simulink model "UDP_INTEGRATION_TEST_01"  (Simulink 8.1)
settings: Solver=ode4  StartTime=0.0  StopTime=inf  FixedStep=Ts  MaxStep=1e-3  RelTol=1e-3
model workspace (MAT data in the model file):
  op_snapshot1 : opcond.OperatingPoint (value not decoded)
PostLoadFcn:
  | INTEGRATION_TEST_01_init;
InitFcn:
  | INTEGRATION_TEST_01_init;
undefined symbols (not defined in the file or in its folder): cable_spec, fdesignblkfcn, gcbh, generic_ethernet_cb, Left, relay_par, Ts, type, V
libraries: powerlib_extras x14, rtio_opalrt_common x13, rtlab x10, cables_lib x6, breaker_lib x4, simulink_extras x4, simulink x4, Load_lib x3, rtio_generic_modbus x3, powerlib x2, ssn_lib x2, transformer_lib x2
(part 1 of 2)
settings Model: ARTEMISmethode_block_infos=$$__separator__$$UDP_INTEGRATION_TEST_01/ARTEMIS Guide$$__separator__$$  Creator=RE25624  LastModifiedBy=re25624  BufferReuse=off
settings SolverCC: ZeroCrossAlgorithm=Adaptive
settings DataIOCC: ExternalInput=getinputstruct(op_snapshot1)  InitialState=getstatestruct(op_snapshot1)  LimitDataPoints=off  MaxDataPoints=90060  SignalLoggingSaveFormat=Dataset  SaveOutput=off  SignalLogging=off  DSMLogging=off  SaveTime=off  OutputSaveName=result
settings OptimizationCC: BlockReduction=off  OptimizeBlockIOStorage=off  BufferReuse=off  ExpressionFolding=off  LocalBlockOutputs=off
settings DebuggingCC: MaxConsecutiveZCsMsg=warning  IgnoredZcDiagnostic=none  SolverPrmCheckMsg=none  MultiTaskRateTransMsg=warning  FcnCallInpInsideContextMsg=EnableAllAsWarning  FrameProcessingCompatibilityMsg=error  ModelReferenceExtraNoncontSigs=warning  StrictBusMsg=None
settings ModelReferenceCC: UpdateModelReferenceTargets=IfOutOfDate
settings SFSimCC: SFSimEcho=off
settings GRTTargetCC: CodeReplacementLibrary=C89/C90 (ANSI)

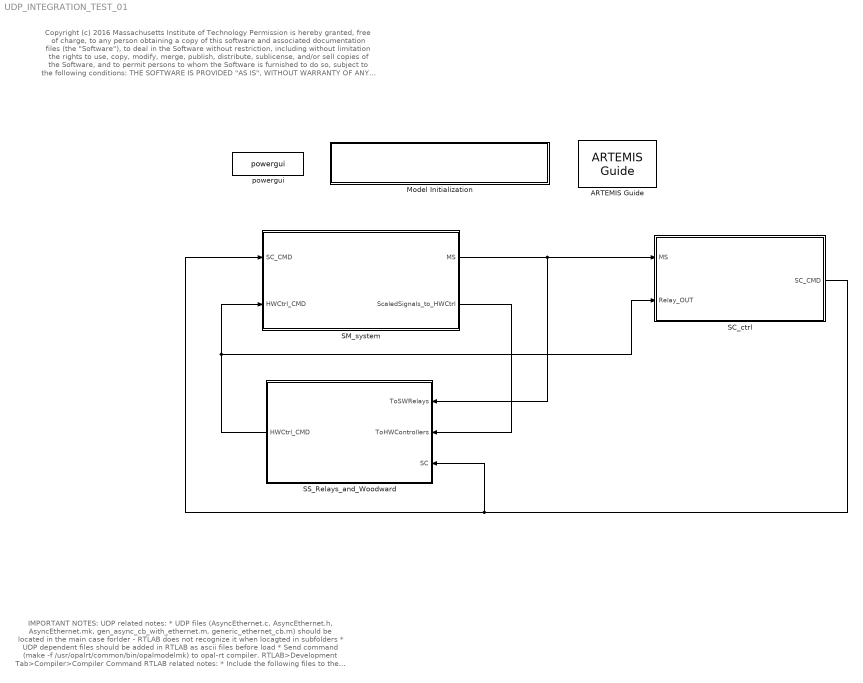
== system UDP_INTEGRATION_TEST_01 ==
  note: Copyright (c) 2016 Massachusetts Institute of Technology
      | Permission is hereby granted, free of charge, to any person obtaining a copy of this software and associated documentation files (the "Software"), to deal
      | in the Software without restriction, including without limitation the rights to use, copy, modify, merge, publish, distribute, sublicense, and/or sell copies of the
      | Software, and to permit persons to whom the Software is furnished to do so, subject to the following conditions:
      |
      | THE SOFTWARE IS PROVIDED "AS IS", WITHOUT WARRANTY OF ANY KIND, EXPRESS OR IMPLIED, INCLUDING BUT NOT LIMITED TO THE
      | WARRANTIES OF MERCHANTABILITY, FITNESS FOR A PARTICULAR PURPOSE AND NONINFRINGEMENT. IN NO EVENT SHALL THE AUTHORS
      | OR COPYRIGHT HOLDERS BE LIABLE FOR ANY CLAIM, DAMAGES OR OTHER LIABILITY, WHETHER IN AN ACTION OF CONTRACT, TORT OR
      | OTHERWISE, ARISING FROM, OUT OF OR IN CONNECTION WITH THE SOFTWARE OR THE USE OR OTHER DEALINGS IN THE SOFTWARE.
  note: IMPORTANT NOTES:
      |
      | UDP related notes:
      | * UDP files (AsyncEthernet.c, AsyncEthernet.h, AsyncEthernet.mk, gen_async_cb_with_ethernet.m, generic_ethernet_cb.m)
      | should be located in the main case forlder - RTLAB does not recognize it when locagted in subfolders
      | * UDP dependent files should be added in RTLAB as ascii files before load
      | * Send command (make -f /usr/opalrt/common/bin/opalmodelmk) to opal-rt compiler.   RTLAB>Development Tab>Compiler>Compiler Command
      |
      | RTLAB related notes:
      | * Include the following files to the case before compilation:
      | ascii (..\..\..\..\..\Program Files (x86)\MATLAB\R2013a\toolbox\physmod\powersys\powersys\sfun_discreteVariableDelay.c)
      | binary (..\..\..\..\..\Program Files (x86)\MATLAB\R2013a\toolbox\physmod\powersys\powersys\sfun_discreteVariableDelay.mexw32)
  ARTEMIS Guide : artemis/ARTEMIS/ARTEMIS Guide  Tag=FTSSmethode_opal_4hx0r99  Description=5.0_z1  lock=on  Ts=Ts  opt=art5  dyna=off  nb_perm=4  RT_fullcomp=off  ssn=on  ssn_itvc=off  ssn_ivic=off  ssn_ext=off  ssn_solver=Art5 with Backward Euler nodal interface  ssn_impulse=off  ssn_quasimpulse=off  ssn_impulse_loop=2  paraExtinctionThy=off  Thy_Impulse=on  dtc=Off  dtc_opt=normal  ao=on  simtype=off  ct_mac=off  lin_mov=off  lsp=[0.001 2]  spike_skip=Disabled  dtc_extra=1  dtc_sws=normal  dtc_pied=0.5  SPSRulesBlock=SPSRules  tre=on  ctmm=off  LF=off  dpl_type=ARTEMiS DPL  rlc_type=off  custom_type=off  para=on  ssn_ImpulseLoopBlockedStateUpdate=2  ssn_mov_iter_number=5  ssn_switch_iter_number=5
  Model Initialization : Subsystem  AncestorBlock=artemis/Tools /Misc/Model Initialization  mask(Model Functions){InitFcnX=INTEGRATION_TEST_01_init;, prel=off, posl=on, inif=on, strf=off}
      mask prompts: InitFcnX "Initialisation"; prel "Preload Function"; posl "PostLoad Function"; inif "InitFcn"; strf "StartFcn"
      mask init:
      | currentBlock = gcb;
      | root = bdroot(currentBlock);
      | 
      | 
      | if ~strcmp(get_param(root,'BlockDiagramType'),'library')
      |     if prel==1
      |         set_param(root, 'PreLoadFcn', InitFcnX);
      |     else
      |         set_param(root, 'PreLoadFcn', '');
      |     end
      |     if inif==1
      |         set_param(root, 'InitFcn', InitFcnX);
      |     else
      |         set_param(root, 'InitFcn', '');
      |     end
      |     if strf==1
      |         set_param(root, 'StartFcn', InitFcnX);
      |     else
      |         set_param(root, 'StartFcn', '');
      |     end
      |     if posl==1
      |         set_param(root, 'PostLoadFcn', InitFcnX);
      |     else
      |         set_param(root, 'PostLoadFcn', '');
      |     end
      | end
      | 
      | pos = get_param(currentBlock, 'Position');
      | width = pos(3) - pos(1); height = pos(4) - pos(2);
      | txt = [ upper(root) '\n' '- InitFcn. . . . . '  get_param(root, 'InitFcn') ];
      settings: CopyFcn=set_param(gcb,'LinkStatus','inactive')
      mask Display: text(5, height*0.5, txt, 'horizontalAlignment', 'left', 'verticalAlignment', 'middle') ;
  SC_ctrl : Subsystem
  SM_system : Subsystem
  SS_Relays_and_Woodward : Subsystem
  powergui : powerlib/powergui  Priority=2  SimulationMode=Discrete  SolverType=Tustin  SampleTime=Ts  frequency=60  SPID=off  DisableSnubberDevices=off  DisableRonSwitches=off  DisableVfSwitches=off  SwTol=0  Interpol=off  DisplayEquations=off  frequencyindice=0  Pbase=100e6  ErrMax=1e-4  Iterations=50  UnitsV=kV  UnitsW=MW  FunctionMessages=off  echomessages=off  HookPort=off  EnableUseOfTLC=off  x0status=blocks  RestoreLinks=warning  ResistiveCurrentMeasurement=off  Frange=logspace(0,3,50)  Ylog=off  Xlog=off  ShowGrid=off  save=off  variable=ZData  structure=0  ZoomFFT=on  StartTime=0.0  cycles=2  DisplayStyle=off  fundamental=60  FreqAxis=off  MaxFrequency=1000  frequencyindicesteady=1  RmsSteady=1  display=off  Ts=0  methode=off
  wires:
  SS_Relays_and_Woodward/1(HWCtrl_CMD) -> SM_system/2(HWCtrl_CMD), SC_ctrl/2(Relay_OUT)
  SC_ctrl/1(SC_CMD) -> SS_Relays_and_Woodward/3(SC), SM_system/1(SC_CMD)
  SM_system/1(MS) -> SC_ctrl/1(MS), SS_Relays_and_Woodward/1(ToSWRelays)
  SM_system/2(ScaledSignals_to_HWCtrl) -> SS_Relays_and_Woodward/2(ToHWControllers)

== system UDP_INTEGRATION_TEST_01/Model Initialization ==

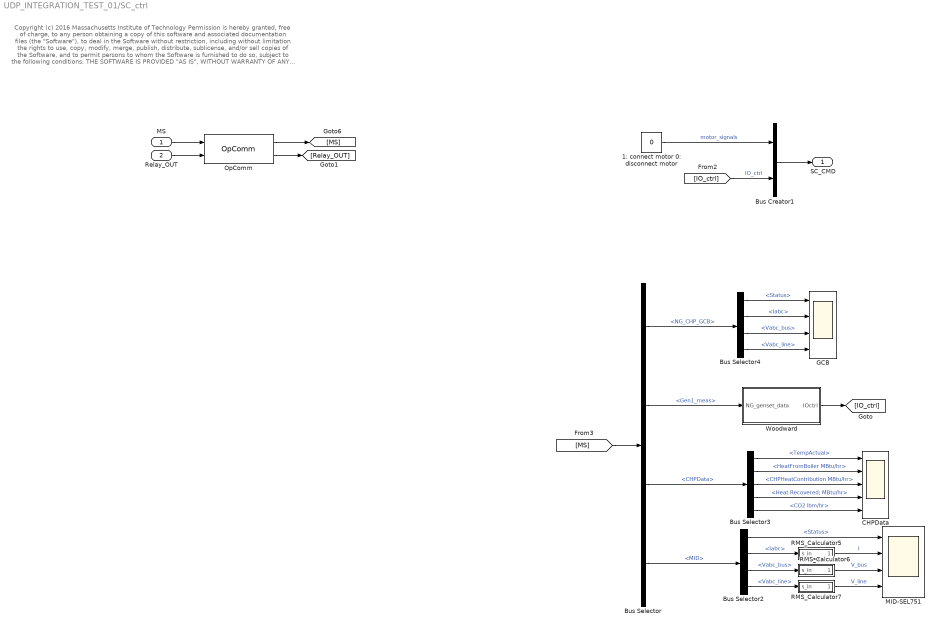
== system UDP_INTEGRATION_TEST_01/SC_ctrl ==
  note: Copyright (c) 2016 Massachusetts Institute of Technology
      | Permission is hereby granted, free of charge, to any person obtaining a copy of this software and associated documentation files (the "Software"), to deal
      | in the Software without restriction, including without limitation the rights to use, copy, modify, merge, publish, distribute, sublicense, and/or sell copies of the
      | Software, and to permit persons to whom the Software is furnished to do so, subject to the following conditions:
      |
      | THE SOFTWARE IS PROVIDED "AS IS", WITHOUT WARRANTY OF ANY KIND, EXPRESS OR IMPLIED, INCLUDING BUT NOT LIMITED TO THE
      | WARRANTIES OF MERCHANTABILITY, FITNESS FOR A PARTICULAR PURPOSE AND NONINFRINGEMENT. IN NO EVENT SHALL THE AUTHORS
      | OR COPYRIGHT HOLDERS BE LIABLE FOR ANY CLAIM, DAMAGES OR OTHER LIABILITY, WHETHER IN AN ACTION OF CONTRACT, TORT OR
      | OTHERWISE, ARISING FROM, OUT OF OR IN CONNECTION WITH THE SOFTWARE OR THE USE OR OTHER DEALINGS IN THE SOFTWARE
  MS : Inport
  Relay_OUT : Inport  Port=2
  1: connect motor 0: disconnect motor : Constant  Value=0
  Bus Creator1 : BusCreator  Inputs=2
  Bus Selector : BusSelector  OutputSignals=NG_CHP_MS.NG_CHP_GCB,NG_CHP_MS.Gen1_meas,NG_CHP_MS.CHPData,MID
  Bus Selector2 : BusSelector  OutputSignals=Status,Iabc,Vabc_bus,Vabc_line
  Bus Selector3 : BusSelector  OutputSignals=TempActual,HeatFromBoiler MBtu/hr,CHPHeatContribution MBtu/hr,Thermal data.Heat Recovered; MBtu/hr,Thermal data.CO2 lbm/hr
  Bus Selector4 : BusSelector  OutputSignals=Status,Iabc,Vabc_bus,Vabc_line
  CHPData : Scope  NumInputPorts=5
      settings: ShowLegends=on  TimeRange=10  YMin=19.11~0~-1~1.37518~932.98  YMax=19.2~5.5~1~1.37533~933.08  SaveName=ScopeData3
  GCB : Scope  NumInputPorts=4
      settings: ShowLegends=on  TimeRange=1  YMin=-1~-0.001~-12000~-12000  YMax=1~0.001~12000~12000  SaveName=ScopeData6
  MID-SEL751 : Scope  NumInputPorts=4
      settings: ShowLegends=on  TimeRange=1  YMin=0.95~-225~-12000~-12000  YMax=1.05~225~12000~12000  SaveName=ScopeData9
  OpComm : rtlab/OpComm  nbport=2  groupe_acq=1  subsys_rate=0  st=0  Synchronization=on  Interpolation=on  Threshold=1.0  Missed_Data=off  Sim_Time=off  Samples=off  dynSigOut=off  from_console=0  warning_done=off  writeOpCommFile=off  Offset=off
  RMS_Calculator5 : Subsystem
  RMS_Calculator6 : Subsystem
  RMS_Calculator7 : Subsystem
  Woodward : Subsystem
  SC_CMD : Outport
  wires:
  OpComm/1 -> [MS]
  MS/1 -> OpComm/1
  OpComm/2 -> [Relay_OUT]
  Relay_OUT/1 -> OpComm/2
  [IO_ctrl] -> Bus Creator1/2  "IO_ctrl"
  1: connect motor 0: disconnect motor/1 -> Bus Creator1/1  "motor_signals"
  Bus Creator1/1 -> SC_CMD/1
  Bus Selector/4 -> Bus Selector2/1  "<MID>"
  RMS_Calculator7/1(s_out) -> MID-SEL751/4  "V_line"
  RMS_Calculator6/1(s_out) -> MID-SEL751/3  "V_bus"
  RMS_Calculator5/1(s_out) -> MID-SEL751/2  "I"
  Bus Selector2/4 -> RMS_Calculator7/1(s_in)  "<Vabc_line>"
  Bus Selector2/3 -> RMS_Calculator6/1(s_in)  "<Vabc_bus>"
  Bus Selector2/2 -> RMS_Calculator5/1(s_in)  "<Iabc>"
  Bus Selector2/1 -> MID-SEL751/1  "<Status>"
  Bus Selector3/4 -> CHPData/4  "<Heat Recovered; MBtu/hr>"
  Bus Selector3/3 -> CHPData/3  "<CHPHeatContribution MBtu/hr>"
  Bus Selector3/2 -> CHPData/2  "<HeatFromBoiler MBtu/hr>"
  Bus Selector3/5 -> CHPData/5  "<CO2 lbm/hr>"
  Bus Selector3/1 -> CHPData/1  "<TempActual>"
  Bus Selector/3 -> Bus Selector3/1  "<CHPData>"
  [MS] -> Bus Selector/1
  Bus Selector/2 -> Woodward/1(NG_genset_data)  "<Gen1_meas>"
  Bus Selector/1 -> Bus Selector4/1  "<NG_CHP_GCB>"
  Bus Selector4/4 -> GCB/4  "<Vabc_line>"
  Bus Selector4/3 -> GCB/3  "<Vabc_bus>"
  Bus Selector4/2 -> GCB/2  "<Iabc>"
  Bus Selector4/1 -> GCB/1  "<Status>"
  Woodward/1(IOctrl) -> [IO_ctrl]

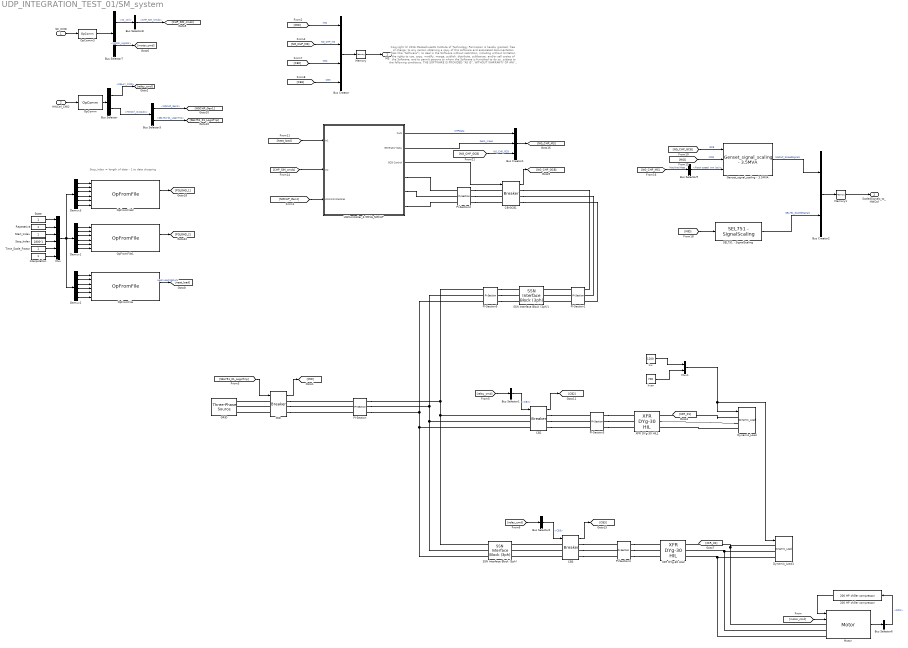
== system UDP_INTEGRATION_TEST_01/SM_system ==
  note: Copyright (c) 2016 Massachusetts Institute of Technology
      | Permission is hereby granted, free of charge, to any person obtaining a copy of this software and associated documentation files (the "Software"), to deal
      | in the Software without restriction, including without limitation the rights to use, copy, modify, merge, publish, distribute, sublicense, and/or sell copies of the
      | Software, and to permit persons to whom the Software is furnished to do so, subject to the following conditions:
      |
      | THE SOFTWARE IS PROVIDED "AS IS", WITHOUT WARRANTY OF ANY KIND, EXPRESS OR IMPLIED, INCLUDING BUT NOT LIMITED TO THE
      | WARRANTIES OF MERCHANTABILITY, FITNESS FOR A PARTICULAR PURPOSE AND NONINFRINGEMENT. IN NO EVENT SHALL THE AUTHORS
      | OR COPYRIGHT HOLDERS BE LIABLE FOR ANY CLAIM, DAMAGES OR OTHER LIABILITY, WHETHER IN AN ACTION OF CONTRACT, TORT OR
      | OTHERWISE, ARISING FROM, OUT OF OR IN CONNECTION WITH THE SOFTWARE OR THE USE OR OTHER DEALINGS IN THE SOFTWARE
  note: Stop_index = length of data - 1 to data chopping
  SC_CMD : Inport
  HWCtrl_CMD : Inport  Port=2
  200 HP chiller compressor : Load_lib/200 HP chiller compressor
  Bus Creator : BusCreator
  Bus Creator1 : BusCreator  Inputs=3
  Bus Creator2 : BusCreator  Inputs=2
  Bus Selector : BusSelector  OutputSignals=RELAY_CMD,HWCtrl_Outputs
  Bus Selector1 : BusSelector  OutputSignals=CB2
  Bus Selector2 : BusSelector  OutputSignals=CB3
  Bus Selector3 : BusSelector  OutputSignals=NGCHP_Gen1,SEL751-01_LogicTrip
  Bus Selector6 : BusSelector  OutputSignals=RPM
  Bus Selector7 : BusSelector  OutputSignals=IO_ctrl,motor_signals
  Bus Selector8 : BusSelector  OutputSignals=16 DOUT GR3.CHP_SIM_Cmds
  Bus Selector9 : BusSelector  OutputSignals="Gen1_meas.w.w.Rotor speed  wm (pu)"
  CB-GCB1 : breaker_lib/Breaker  Ts=Ts  mech_delay=cb_mech_delay
  CB2 : breaker_lib/Breaker  Ts=Ts  mech_delay=cb_mech_delay
  CB3 : breaker_lib/Breaker  Ts=Ts  mech_delay=cb_mech_delay
  Demux1 : Demux  Outputs=6
  Demux2 : Demux  Outputs=6
  Demux3 : Demux  Outputs=6
  Dynamic_Load : Load_lib/Dynamic_Load  V=480  Ts=Ts
  Dynamic_Load1 : Load_lib/Dynamic_Load  V=480  Ts=Ts
  GRID : powerlib/Electrical Sources/Three-Phase Source  Voltage=13800  PhaseAngle=0  Frequency=60  InternalConnection=Yg  SpecifyImpedance=on  Resistance=0.8929  Inductance=16.58e-3  ShortCircuitLevel=375e6  BaseVoltage=13800  XRratio=4.6  BusType=swing  Pref=0  Qref=0  Qmin=-inf  Qmax=inf
  Genset_signal_scaling - 3.5MVA : EasyGen3500_GensetSignalScaling_lib/Genset_signal_scaling - 3.5MVA  Vpk_mcb=11268  watt_mcb=3150000  Vpk_gcb=11268  watt_gcb=3150000  rated_rpm=1800  wm_noise_bias=0.02
  HWController_3.5MVA_NGCHP : Subsystem  AncestorBlock=HWController_NGCHP_Genset_3p5MVA_lib/HWController_3.5MVA_NGCHP
  "Interpolation " : Constant
  MID : breaker_lib/Breaker  Ts=Ts  mech_delay=cb_mech_delay
  Memory : Memory
  Memory1 : Memory
  Motor : Motor_InductionMachine_lib/Motor
  Mux : Mux  Inputs=6
  Mux1 : Mux  Inputs=2
  OpComm : rtlab/OpComm  nbport=1  groupe_acq=1  subsys_rate=0  st=0  Synchronization=on  Interpolation=on  Threshold=1.0  Missed_Data=off  Sim_Time=off  Samples=off  dynSigOut=off  from_console=0  warning_done=off  writeOpCommFile=off  Offset=off
  OpComm3 : rtlab/OpComm  nbport=1  groupe_acq=1  subsys_rate=0  st=0  Synchronization=on  Interpolation=on  Threshold=1.0  Missed_Data=off  Sim_Time=off  Samples=off  dynSigOut=off  from_console=1  warning_done=off  writeOpCommFile=off  Offset=off
  OpFromFile : rtlab/DataLogging/OpFromFile  filename_mode=Static (same filename all the time)  reload_mode=Next time model is paused (Real-Time)  init_file_id=0  filename=HeatLoad.mat  rtpath='./'  nrtpath='.\'  sample_time=Ts
  OpFromFile1 : rtlab/DataLogging/OpFromFile  filename_mode=Static (same filename all the time)  reload_mode=Next time model is paused (Real-Time)  init_file_id=0  filename=one_min_data.mat  rtpath='./'  nrtpath='.\'  sample_time=0
  OpFromFile2 : rtlab/DataLogging/OpFromFile  filename_mode=Static (same filename all the time)  reload_mode=Next time model is paused (Real-Time)  init_file_id=0  filename=one_min_data.mat  rtpath='./'  nrtpath='.\'  sample_time=0
  PI-Section : cables_lib/PI-Section  cable_spec=[cable_spec(13, :)]  line_length=5500  parallel_sets=2
  PI-Section1 : cables_lib/PI-Section  cable_spec=[cable_spec(11, :)]  line_length=10  parallel_sets=1
  PI-Section2 : cables_lib/PI-Section  cable_spec=[cable_spec(11, :)]  line_length=2000  parallel_sets=1
  PI-Section3 : cables_lib/PI-Section  cable_spec=[cable_spec(13, :)]  line_length=1500  parallel_sets=1
  PI-Section4 : cables_lib/PI-Section  cable_spec=[cable_spec(13, :)]  line_length=2000  parallel_sets=2
  PI-Section5 : cables_lib/PI-Section  cable_spec=[cable_spec(11, :)]  line_length=10  parallel_sets=1
  "Repetative " : Constant
  SEL751 - SignalScaling : SEL751_SignalScaling_lib/SEL751 - SignalScaling  ct_ratio=1/1250  pt_ratio=1/1800
  SSN Interface Block (3ph) : ssn_lib/SSN Interface Block (3ph)  nb_phase=3  nb_port=2  p1_type=V-type(Left)  p2_type=V-type (Right)  p3_type=V-type(Left)  p4_type=V-type(Left)  p5_type=V-type(Left)  p6_type=V-type(Left)  p7_type=V-type(Left)  p8_type=V-type(Left)  p9_type=V-type(Left)  p10_type=V-type(Left)  p11_type=V-type(Left)  p12_type=V-type(Left)  p13_type=V-type(Left)  p14_type=V-type(Left)  p15_type=V-type(Left)  p16_type=V-type(Left)  I_port_shunt_resistance=1e9
  SSN Interface Block (3ph)1 : ssn_lib/SSN Interface Block (3ph)  nb_phase=3  nb_port=2  p1_type=V-type(Left)  p2_type=V-type (Right)  p3_type=V-type(Left)  p4_type=V-type(Left)  p5_type=V-type(Left)  p6_type=V-type(Left)  p7_type=V-type(Left)  p8_type=V-type(Left)  p9_type=V-type(Left)  p10_type=V-type(Left)  p11_type=V-type(Left)  p12_type=V-type(Left)  p13_type=V-type(Left)  p14_type=V-type(Left)  p15_type=V-type(Left)  p16_type=V-type(Left)  I_port_shunt_resistance=1e9
  "Start_Index " : Constant
  "State " : Constant
  "Stop_Index " : Constant  Value=1800-1
  "Time_Scale_Factor " : Constant
  XFR DYg-30 HIL1 : transformer_lib/XFR DYg-30 HIL  Rating=2500  Vp=13800  Vs=480  Z=5.75  XR=6.6
  XFR DYg-30 HIL2 : transformer_lib/XFR DYg-30 HIL  Rating=2500  Vp=13800  Vs=480  Z=5.75  XR=6.6
  kvar : Constant  Value=700
  kw : Constant  Value=1200
  MS : Outport
  ScaledSignals_to_HWCtrl : Outport  Port=2
  wires:
  MID/1 -> [MID]
  ? -> [XFR_01]
  "Stop_Index "/1 -> Mux/4
  Demux1/2 -> OpFromFile1/2
  Demux1/5 -> OpFromFile1/5
  OpFromFile1/2 -> [PQLOAD_2]
  "Interpolation "/1 -> Mux/6
  Demux1/4 -> OpFromFile1/4
  Demux1/1 -> OpFromFile1/1
  Demux1/6 -> OpFromFile1/6
  Demux1/3 -> OpFromFile1/3
  "Start_Index "/1 -> Mux/3
  "Time_Scale_Factor "/1 -> Mux/5
  "Repetative "/1 -> Mux/2
  "State "/1 -> Mux/1
  OpFromFile/2 -> [heat_load]  "Heat Load MBtu/hr"
  Demux2/2 -> OpFromFile/2
  Demux2/5 -> OpFromFile/5
  Demux2/4 -> OpFromFile/4
  Demux2/1 -> OpFromFile/1
  Demux2/6 -> OpFromFile/6
  Demux2/3 -> OpFromFile/3
  ? -> [XFR_02]
  CB2/1 -> [CB2]
  CB3/1 -> [CB3]
  Demux3/2 -> OpFromFile2/2
  Demux3/5 -> OpFromFile2/5
  OpFromFile2/2 -> [PQLOAD_1]
  Demux3/4 -> OpFromFile2/4
  Demux3/1 -> OpFromFile2/1
  Demux3/6 -> OpFromFile2/6
  Demux3/3 -> OpFromFile2/3
  Mux/1 -> Demux3/1, Demux2/1, Demux1/1
  [relay_cmd] -> Bus Selector1/1
  Bus Selector1/1 -> CB2/1  "<CB2>"
  [relay_cmd] -> Bus Selector2/1
  Bus Selector2/1 -> CB3/1  "<CB3>"
  [SEL751_01_LogicTrip] -> MID/1
  [motor_cmd] -> Motor/2
  Motor/1 -> Bus Selector6/1
  Bus Selector6/1 -> 200 HP chiller compressor/1  "<RPM>"
  200 HP chiller compressor/1 -> Motor/1
  CB-GCB1/1 -> [NG_CHP_GCB]
  [NG_CHP_GCB] -> Bus Creator1/3  "NG_CHP_GCB"
  HWController_3.5MVA_NGCHP/2(Generator Data) -> Bus Creator1/2  "Gen1_meas"
  HWController_3.5MVA_NGCHP/1(Out1) -> Bus Creator1/1  "CHPData"
  [heat_load] -> HWController_3.5MVA_NGCHP/1(In1)
  [CHP_SIM_cmds] -> HWController_3.5MVA_NGCHP/2(In2)
  Bus Creator1/1 -> [NG_CHP_MS]
  [NGCHP_Gen1] -> HWController_3.5MVA_NGCHP/3(HWControllerBias)
  HWController_3.5MVA_NGCHP/3(GCB Control) -> CB-GCB1/1
  Bus Creator/1 -> Memory/1
  SC_CMD/1 -> OpComm3/1
  Bus Selector8/1 -> [CHP_SIM_cmds]  "<CHP_SIM_Cmds>"
  [MID] -> Bus Creator/1  "MID"
  [NG_CHP_MS] -> Bus Creator/2  "NG_CHP_MS"
  OpComm3/1 -> Bus Selector7/1
  Bus Selector7/1 -> Bus Selector8/1  "<IO_ctrl>"
  Memory/1 -> MS/1
  HWCtrl_CMD/1 -> OpComm/1
  [NG_CHP_MS] -> Bus Selector9/1  "Machine Meas"
  [NG_CHP_GCB] -> Genset_signal_scaling - 3.5MVA/1  "GCB"
  [MID] -> Genset_signal_scaling - 3.5MVA/2  "MCB"
  Bus Selector9/1 -> Genset_signal_scaling - 3.5MVA/3  "<Rotor speed  wm (pu)>"
  Bus Creator2/1 -> Memory1/1
  Memory1/1 -> ScaledSignals_to_HWCtrl/1
  Genset_signal_scaling - 3.5MVA/1 -> Bus Creator2/1  "NGCHP_ScaledSignals"
  [CB2] -> Bus Creator/3  "CB2"
  [CB3] -> Bus Creator/4  "CB3"
  Bus Selector7/2 -> [motor_cmd]  "<motor_signals>"
  SEL751 - SignalScaling/1 -> Bus Creator2/2  "SEL751_ScaledSignals"
  [MID] -> SEL751 - SignalScaling/1
  Bus Selector3/1 -> [NGCHP_Gen1]  "<NGCHP_Gen1>"
  Bus Selector3/2 -> [SEL751_01_LogicTrip]  "<SEL751-01_LogicTrip>"
  OpComm/1 -> Bus Selector/1
  Bus Selector/1 -> [relay_cmd]  "<RELAY_CMD>"
  Bus Selector/2 -> Bus Selector3/1  "<HWCtrl_Outputs>"
  Mux1/1 -> Dynamic_Load/1, Dynamic_Load1/1
  kw/1 -> Mux1/1
  kvar/1 -> Mux1/2
  connections:
  CB2/RConn2 -- PI-Section3/LConn2
  CB2/RConn1 -- PI-Section3/LConn1
  CB2/RConn3 -- PI-Section3/LConn3
  CB3/RConn2 -- PI-Section4/LConn2
  CB3/RConn1 -- PI-Section4/LConn1
  CB3/RConn3 -- PI-Section4/LConn3
  CB3/LConn2 -- SSN Interface Block (3ph)/RConn2
  CB3/LConn1 -- SSN Interface Block (3ph)/RConn1
  CB3/LConn3 -- SSN Interface Block (3ph)/RConn3
  PI-Section5/LConn3 -- PI-Section/RConn3 -- SSN Interface Block (3ph)/LConn3 -- CB2/LConn3
  PI-Section5/LConn2 -- PI-Section/RConn2 -- SSN Interface Block (3ph)/LConn2 -- CB2/LConn2
  PI-Section5/LConn1 -- PI-Section/RConn1 -- SSN Interface Block (3ph)/LConn1 -- CB2/LConn1
  Motor/LConn1 -- Dynamic_Load1/LConn1 -- XFR DYg-30 HIL2/RConn1
  Motor/LConn3 -- Dynamic_Load1/LConn3 -- XFR DYg-30 HIL2/RConn3
  Motor/LConn2 -- XFR DYg-30 HIL2/RConn2 -- Dynamic_Load1/LConn2
  PI-Section4/RConn1 -- XFR DYg-30 HIL2/LConn1
  PI-Section4/RConn2 -- XFR DYg-30 HIL2/LConn2
  PI-Section4/RConn3 -- XFR DYg-30 HIL2/LConn3
  PI-Section3/RConn2 -- XFR DYg-30 HIL1/LConn2
  PI-Section3/RConn3 -- XFR DYg-30 HIL1/LConn3
  PI-Section3/RConn1 -- XFR DYg-30 HIL1/LConn1
  PI-Section1/LConn1 -- SSN Interface Block (3ph)1/RConn1
  PI-Section1/LConn2 -- SSN Interface Block (3ph)1/RConn2
  PI-Section1/LConn3 -- SSN Interface Block (3ph)1/RConn3
  PI-Section5/RConn2 -- SSN Interface Block (3ph)1/LConn2
  PI-Section5/RConn1 -- SSN Interface Block (3ph)1/LConn1
  PI-Section5/RConn3 -- SSN Interface Block (3ph)1/LConn3
  MID/RConn3 -- PI-Section/LConn3
  MID/RConn2 -- PI-Section/LConn2
  MID/RConn1 -- PI-Section/LConn1
  MID/LConn3 -- GRID/RConn3
  MID/LConn1 -- GRID/RConn1
  MID/LConn2 -- GRID/RConn2
  HWController_3.5MVA_NGCHP/RConn2 -- PI-Section2/LConn2
  PI-Section2/RConn1 -- CB-GCB1/LConn1
  PI-Section2/RConn2 -- CB-GCB1/LConn2
  PI-Section2/RConn3 -- CB-GCB1/LConn3
  HWController_3.5MVA_NGCHP/RConn1 -- PI-Section2/LConn1
  HWController_3.5MVA_NGCHP/RConn3 -- PI-Section2/LConn3
  CB-GCB1/RConn1 -- PI-Section1/RConn1
  CB-GCB1/RConn2 -- PI-Section1/RConn2
  CB-GCB1/RConn3 -- PI-Section1/RConn3
  Dynamic_Load/LConn2 -- XFR DYg-30 HIL1/RConn2
  Dynamic_Load/LConn3 -- XFR DYg-30 HIL1/RConn3
  Dynamic_Load/LConn1 -- XFR DYg-30 HIL1/RConn1

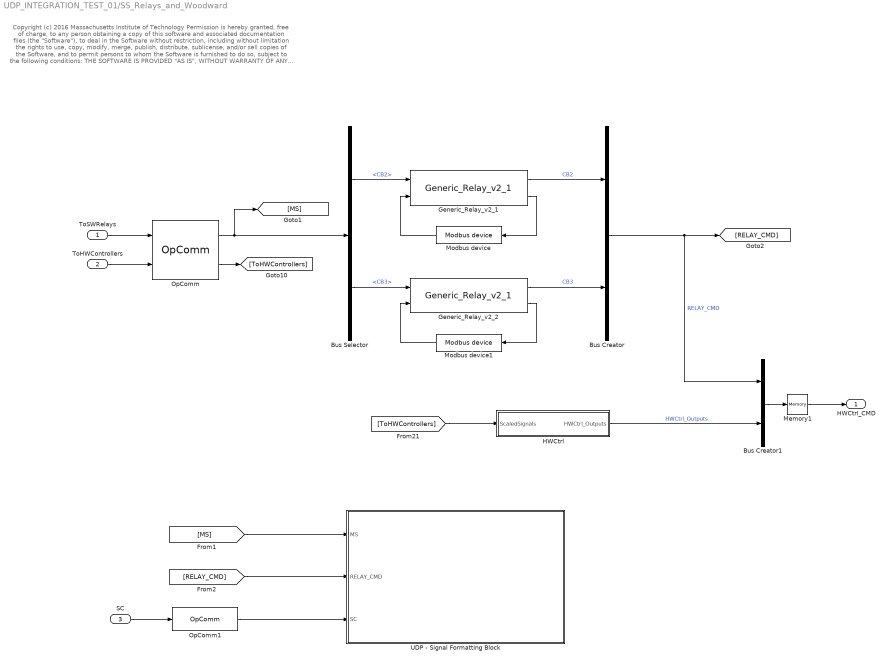
== system UDP_INTEGRATION_TEST_01/SS_Relays_and_Woodward ==
  note: Copyright (c) 2016 Massachusetts Institute of Technology
      | Permission is hereby granted, free of charge, to any person obtaining a copy of this software and associated documentation files (the "Software"), to deal
      | in the Software without restriction, including without limitation the rights to use, copy, modify, merge, publish, distribute, sublicense, and/or sell copies of the
      | Software, and to permit persons to whom the Software is furnished to do so, subject to the following conditions:
      |
      | THE SOFTWARE IS PROVIDED "AS IS", WITHOUT WARRANTY OF ANY KIND, EXPRESS OR IMPLIED, INCLUDING BUT NOT LIMITED TO THE
      | WARRANTIES OF MERCHANTABILITY, FITNESS FOR A PARTICULAR PURPOSE AND NONINFRINGEMENT. IN NO EVENT SHALL THE AUTHORS
      | OR COPYRIGHT HOLDERS BE LIABLE FOR ANY CLAIM, DAMAGES OR OTHER LIABILITY, WHETHER IN AN ACTION OF CONTRACT, TORT OR
      | OTHERWISE, ARISING FROM, OUT OF OR IN CONNECTION WITH THE SOFTWARE OR THE USE OR OTHER DEALINGS IN THE SOFTWARE
  ToSWRelays : Inport
  ToHWControllers : Inport  Port=2
  SC : Inport  Port=3
  Bus Creator : BusCreator  Inputs=2
  Bus Creator1 : BusCreator  Inputs=2
  Bus Selector : BusSelector  OutputSignals=CB2,CB3
  Generic_Relay_v2_1 : relay_modbus_lib/Generic_Relay_v2_1  Ts=Ts  relay_settings=[relay_par(1,:)]
  Generic_Relay_v2_2 : relay_modbus_lib/Generic_Relay_v2_1  Ts=Ts  relay_settings=[relay_par(2,:)]
  HWCtrl : Subsystem
  Memory1 : Memory
  Modbus device : rtio_generic_modbus/Modbus device  conf_name=F1_relay_cfg1.opal  conf_name_mask=F1_relay_cfg1.xls  sample_time=Ts
  Modbus device1 : rtio_generic_modbus/Modbus device  conf_name=F1_relay_cfg2.opal  conf_name_mask=F1_relay_cfg2.xls  sample_time=Ts
  OpComm : rtlab/OpComm  nbport=2  groupe_acq=1  subsys_rate=0  st=0  Synchronization=on  Interpolation=on  Threshold=1.0  Missed_Data=off  Sim_Time=off  Samples=off  dynSigOut=off  from_console=0  warning_done=off  writeOpCommFile=off  Offset=off
  OpComm1 : rtlab/OpComm  nbport=1  groupe_acq=1  subsys_rate=0  st=0  Synchronization=on  Interpolation=on  Threshold=1.0  Missed_Data=off  Sim_Time=off  Samples=off  dynSigOut=off  from_console=1  warning_done=off  writeOpCommFile=off  Offset=off
  UDP - Signal Formatting Block : Subsystem
  HWCtrl_CMD : Outport
  wires:
  OpComm/1 -> [MS], Bus Selector/1
  ToSWRelays/1 -> OpComm/1
  Generic_Relay_v2_1/1 -> Bus Creator/1  "CB2"
  Generic_Relay_v2_2/1 -> Bus Creator/2  "CB3"
  Modbus device/1 -> Generic_Relay_v2_1/2
  Generic_Relay_v2_1/2 -> Modbus device/1
  Modbus device1/1 -> Generic_Relay_v2_2/2
  Generic_Relay_v2_2/2 -> Modbus device1/1
  Bus Selector/2 -> Generic_Relay_v2_2/1  "<CB3>"
  Bus Selector/1 -> Generic_Relay_v2_1/1  "<CB2>"
  ToHWControllers/1 -> OpComm/2
  OpComm/2 -> [ToHWControllers]
  [ToHWControllers] -> HWCtrl/1(ScaledSignals)
  Bus Creator1/1 -> Memory1/1
  Bus Creator/1 -> [RELAY_CMD], Bus Creator1/1  "RELAY_CMD"
  Memory1/1 -> HWCtrl_CMD/1
  HWCtrl/1(HWCtrl_Outputs) -> Bus Creator1/2  "HWCtrl_Outputs"
  [MS] -> UDP - Signal Formatting Block/1(MS)
  [RELAY_CMD] -> UDP - Signal Formatting Block/2(RELAY_CMD)
  OpComm1/1 -> UDP - Signal Formatting Block/3(SC)
  SC/1 -> OpComm1/1

== system UDP_INTEGRATION_TEST_01/SC_ctrl/RMS_Calculator5 ==
  s_in : Inport
  Demux : Demux  Outputs=3
  Discrete  Mean value6 : powerlib_extras/Discrete Measurements/Discrete  Mean value  Freq=60  Vinit=0  Ts=Ts
  Mux2 : Mux  Inputs=2
  Product3 : Product  RndMeth=Zero
  Signed Sqrt : Sqrt  SaturateOnIntegerOverflow=on
  s_out : Outport
  wires:
  Demux/1 -> Product3/1, Product3/2
  Product3/1 -> Discrete  Mean value6/1
  Discrete  Mean value6/1 -> Signed Sqrt/1
  s_in/1 -> Mux2/1, Demux/1  "3ph_inst"
  Mux2/1 -> s_out/1  "inst_rms"
  Signed Sqrt/1 -> Mux2/2  "1ph_rms"

== system UDP_INTEGRATION_TEST_01/SC_ctrl/RMS_Calculator6 ==
  s_in : Inport
  Demux : Demux  Outputs=3
  Discrete  Mean value6 : powerlib_extras/Discrete Measurements/Discrete  Mean value  Freq=60  Vinit=0  Ts=Ts
  Mux2 : Mux  Inputs=2
  Product3 : Product  RndMeth=Zero
  Signed Sqrt : Sqrt  SaturateOnIntegerOverflow=on
  s_out : Outport
  wires:
  Demux/1 -> Product3/1, Product3/2
  Product3/1 -> Discrete  Mean value6/1
  Discrete  Mean value6/1 -> Signed Sqrt/1
  s_in/1 -> Mux2/1, Demux/1  "3ph_inst"
  Mux2/1 -> s_out/1  "inst_rms"
  Signed Sqrt/1 -> Mux2/2  "1ph_rms"

== system UDP_INTEGRATION_TEST_01/SC_ctrl/RMS_Calculator7 ==
  s_in : Inport
  Demux : Demux  Outputs=3
  Discrete  Mean value6 : powerlib_extras/Discrete Measurements/Discrete  Mean value  Freq=60  Vinit=0  Ts=Ts
  Mux2 : Mux  Inputs=2
  Product3 : Product  RndMeth=Zero
  Signed Sqrt : Sqrt  SaturateOnIntegerOverflow=on
  s_out : Outport
  wires:
  Demux/1 -> Product3/1, Product3/2
  Product3/1 -> Discrete  Mean value6/1
  Discrete  Mean value6/1 -> Signed Sqrt/1
  s_in/1 -> Mux2/1, Demux/1  "3ph_inst"
  Mux2/1 -> s_out/1  "inst_rms"
  Signed Sqrt/1 -> Mux2/2  "1ph_rms"

== system UDP_INTEGRATION_TEST_01/SC_ctrl/Woodward ==
  NG_genset_data : Inport
  16Din/16Dout GR3 : Subsystem
  Bus Creator2 : BusCreator  Inputs=1
  Bus Creator4 : BusCreator  Inputs=3
  Bus Selector1 : BusSelector  OutputSignals=Pm,Vf,Vt,w
  Bus Selector3 : BusSelector  OutputSignals="wref,w.wood_Gov_bias,w.Rotor speed  wm (pu)"
  NG-CHP : Scope  NumInputPorts=4
      settings: TimeRange=10  YMin=-0.025~-0.5~0~0  YMax=0.45~5.5~1.1~0.425  SaveName=ScopeData4
  Wood_Goiv_bias : Gain  Gain=10
  IOctrl : Outport
  wires:
  Wood_Goiv_bias/1 -> Bus Creator4/2
  Bus Creator4/1 -> NG-CHP/4  "Speed"
  Bus Selector3/3 -> Bus Creator4/3  "<Rotor speed  wm (pu)>"
  Bus Selector3/2 -> Wood_Goiv_bias/1  "<wood_Gov_bias>"
  Bus Selector3/1 -> Bus Creator4/1  "<wref>"
  Bus Selector1/4 -> Bus Selector3/1  "<w>"
  NG_genset_data/1 -> Bus Selector1/1
  Bus Selector1/3 -> NG-CHP/3  "<Vt>"
  Bus Selector1/2 -> NG-CHP/2  "<Vf>"
  Bus Selector1/1 -> NG-CHP/1  "<Pm>"
  Bus Creator2/1 -> IOctrl/1  "IO ctrl"
  16Din/16Dout GR3/1(Dout) -> Bus Creator2/1  "16 DOUT GR3"

== system UDP_INTEGRATION_TEST_01/SM_system/HWController_3.5MVA_NGCHP ==
  note: Copyright (c) 2016 Massachusetts Institute of Technology
      | Permission is hereby granted, free of charge, to any person obtaining a copy of this software and associated documentation files (the "Software"), to deal
      | in the Software without restriction, including without limitation the rights to use, copy, modify, merge, publish, distribute, sublicense, and/or sell copies of the
      | Software, and to permit persons to whom the Software is furnished to do so, subject to the following conditions:
      |
      | THE SOFTWARE IS PROVIDED "AS IS", WITHOUT WARRANTY OF ANY KIND, EXPRESS OR IMPLIED, INCLUDING BUT NOT LIMITED TO THE
      | WARRANTIES OF MERCHANTABILITY, FITNESS FOR A PARTICULAR PURPOSE AND NONINFRINGEMENT. IN NO EVENT SHALL THE AUTHORS
      | OR COPYRIGHT HOLDERS BE LIABLE FOR ANY CLAIM, DAMAGES OR OTHER LIABILITY, WHETHER IN AN ACTION OF CONTRACT, TORT OR
      | OTHERWISE, ARISING FROM, OUT OF OR IN CONNECTION WITH THE SOFTWARE OR THE USE OR OTHER DEALINGS IN THE SOFTWARE
  In1 : Inport
  In2 : Inport  Port=2
  HWControllerBias : Inport  Port=3
  Bus Creator2 : BusCreator
  Bus Selector6 : BusSelector  OutputSignals=Heat Recovered; MBtu/hr
  Bus Selector7 : BusSelector  OutputSignals=TempActual,HeatFromBoiler MBtu/hr,CHPHeatContribution MBtu/hr,Thermal data.Heat Recovered; MBtu/hr,Thermal data.CO2 lbm/hr
  CHPThermalModel : CHP_Model_lib/CHPThermalModel  SIM_HIL=SIM_HIL
  Demux : Demux  Outputs=2
  HWController_NG_Generator : HWController_NGCHP_Genset_3p5MVA_lib/HWController_NG_Generator
  Modbus device : rtio_generic_modbus/Modbus device  conf_name=CHP_slave_cfg.opal  conf_name_mask=CHP_slave_cfg.xls  sample_time=Ts
  Mux1 : Mux  Inputs=5
  A : PMIOPort  Tag=A  Port=1  Side=Right
      settings: AttributesFormatString=A
  B : PMIOPort  Port=2  Side=Right
  C : PMIOPort  Port=3  Side=Right
  Out1 : Outport
  Generator Data : Outport  Port=2
  GCB Control : Outport  Port=3
  wires:
  In2/1 -> CHPThermalModel/5  "CHP_SIM_Cmds"
  Bus Creator2/1 -> Bus Selector7/1, Out1/1  "CHPData"
  Bus Selector6/1 -> CHPThermalModel/1  "<Heat Recovered; MBtu/hr>"
  HWController_NG_Generator/2 -> GCB Control/1
  HWController_NG_Generator/1 -> Generator Data/1
  Modbus device/2 -> Demux/1
  [HeatRec_MBtuhr] -> Bus Selector6/1, Bus Creator2/2  "Thermal data"
  CHPThermalModel/3 -> Bus Creator2/4
  Demux/1 -> CHPThermalModel/3
  Mux1/1 -> Modbus device/4
  In1/1 -> CHPThermalModel/2
  Bus Selector7/1 -> Mux1/1  "<TempActual>"
  Bus Selector7/4 -> Mux1/4  "<Heat Recovered; MBtu/hr>"
  Bus Selector7/5 -> Mux1/5  "<CO2 lbm/hr>"
  Bus Selector7/2 -> Mux1/2  "<HeatFromBoiler MBtu/hr>"
  CHPThermalModel/2 -> Bus Creator2/3
  Demux/2 -> CHPThermalModel/4
  CHPThermalModel/1 -> Bus Creator2/1  "TempActual"
  Bus Selector7/3 -> Mux1/3  "<CHPHeatContribution MBtu/hr>"
  HWController_NG_Generator/3 -> [HeatRec_MBtuhr]  "Thermal data"
  HWControllerBias/1 -> HWController_NG_Generator/1
  connections:
  HWController_NG_Generator/RConn1 -- A/RConn1
  HWController_NG_Generator/RConn2 -- B/RConn1
  HWController_NG_Generator/RConn3 -- C/RConn1

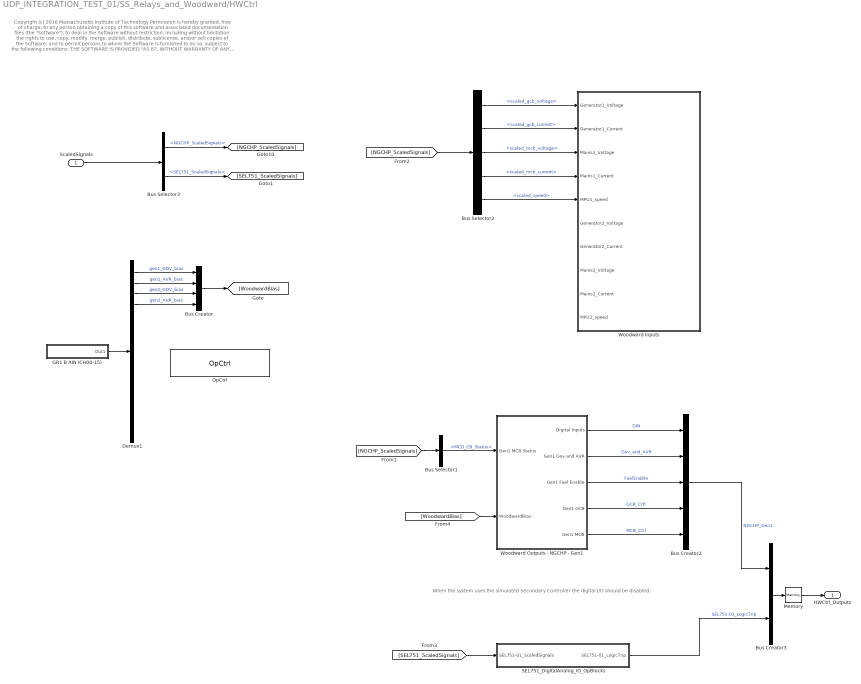
== system UDP_INTEGRATION_TEST_01/SS_Relays_and_Woodward/HWCtrl ==
  note: Copyright (c) 2016 Massachusetts Institute of Technology
      | Permission is hereby granted, free of charge, to any person obtaining a copy of this software and associated documentation files (the "Software"), to deal
      | in the Software without restriction, including without limitation the rights to use, copy, modify, merge, publish, distribute, sublicense, and/or sell copies of the
      | Software, and to permit persons to whom the Software is furnished to do so, subject to the following conditions:
      |
      | THE SOFTWARE IS PROVIDED "AS IS", WITHOUT WARRANTY OF ANY KIND, EXPRESS OR IMPLIED, INCLUDING BUT NOT LIMITED TO THE
      | WARRANTIES OF MERCHANTABILITY, FITNESS FOR A PARTICULAR PURPOSE AND NONINFRINGEMENT. IN NO EVENT SHALL THE AUTHORS
      | OR COPYRIGHT HOLDERS BE LIABLE FOR ANY CLAIM, DAMAGES OR OTHER LIABILITY, WHETHER IN AN ACTION OF CONTRACT, TORT OR
      | OTHERWISE, ARISING FROM, OUT OF OR IN CONNECTION WITH THE SOFTWARE OR THE USE OR OTHER DEALINGS IN THE SOFTWARE
  note: When the system uses the simulated
      | Secondary Controller the digital I/O
      | should be disabled.
  ScaledSignals : Inport
  Bus Creator : BusCreator
  Bus Creator2 : BusCreator  Inputs=5
  Bus Creator3 : BusCreator  Inputs=2
  Bus Selector1 : BusSelector  OutputSignals=MCB_CB_Status
  Bus Selector2 : BusSelector  OutputSignals=scaled_gcb_voltage,scaled_gcb_current,scaled_mcb_voltage,scaled_mcb_current,scaled_speed
  Bus Selector3 : BusSelector  OutputSignals=NGCHP_ScaledSignals,SEL751_ScaledSignals
  Demux1 : Demux  Outputs=16
  GR1 B AIN (CH00-15) : Subsystem
  Memory : Memory
  OpCtrl : rtio_opalrt_common/OpCtrl  CtrlName='OpCtrl'  boardid=0  BitstreamFilename=VC707_2-EX-0001-2_2_6_61-32AIO16DIO16DIOSel-01-01.bin  numconfig=-1  mode=Master  externalClock=off  decimRtsi=0  calibIO=off  SampleTime=0  loadinport=-1  BoardType=VC707  SecondaryPresent=off  sync_type=Audio
  SEL751_DigitalAnalog_IO_OpBlocks : Subsystem
  Woodward Inputs : Subsystem
  Woodward Outputs - NGCHP - Gen1 : Subsystem
  HWCtrl_Outputs : Outport
  wires:
  ScaledSignals/1 -> Bus Selector3/1
  Bus Selector3/1 -> [NGCHP_ScaledSignals]  "<NGCHP_ScaledSignals>"
  Bus Selector3/2 -> [SEL751_ScaledSignals]  "<SEL751_ScaledSignals>"
  [NGCHP_ScaledSignals] -> Bus Selector2/1
  Bus Selector2/5 -> Woodward Inputs/5(MPU1_speed)  "<scaled_speed>"
  Bus Selector2/4 -> Woodward Inputs/4(Mains1_Current)  "<scaled_mcb_current>"
  Bus Selector2/3 -> Woodward Inputs/3(Mains1_Voltage)  "<scaled_mcb_voltage>"
  Bus Selector2/2 -> Woodward Inputs/2(Generator1_Current)  "<scaled_gcb_current>"
  Bus Selector2/1 -> Woodward Inputs/1(Generator1_Voltage)  "<scaled_gcb_voltage>"
  GR1 B AIN (CH00-15)/1(Out1) -> Demux1/1
  Demux1/1 -> Bus Creator/1  "gen1_GOV_bias"
  Demux1/2 -> Bus Creator/2  "gen1_AVR_bias"
  Demux1/3 -> Bus Creator/3  "gen2_GOV_bias"
  Demux1/4 -> Bus Creator/4  "gen2_AVR_bias"
  Bus Creator2/1 -> Bus Creator3/1  "NGCHP_Gen1"
  Woodward Outputs - NGCHP - Gen1/1(Digital Inputs) -> Bus Creator2/1  "DIN"
  Woodward Outputs - NGCHP - Gen1/2(Gen1 Gov and AVR) -> Bus Creator2/2  "Gov_and_AVR"
  Woodward Outputs - NGCHP - Gen1/3(Gen1 Fuel Enable) -> Bus Creator2/3  "FuelEnable"
  Woodward Outputs - NGCHP - Gen1/4(Gen1 GCB) -> Bus Creator2/4  "GCB_Crtl"
  Woodward Outputs - NGCHP - Gen1/5(Gen1 MCB) -> Bus Creator2/5  "MCB_Ctrl"
  [WoodwardBias] -> Woodward Outputs - NGCHP - Gen1/2(WoodwardBias)
  [NGCHP_ScaledSignals] -> Bus Selector1/1
  Bus Selector1/1 -> Woodward Outputs - NGCHP - Gen1/1(Gen1 MCB Status)  "<MCB_CB_Status>"
  Bus Creator3/1 -> Memory/1
  Bus Creator/1 -> [WoodwardBias]
  SEL751_DigitalAnalog_IO_OpBlocks/1(SEL751-01_LogicTrip) -> Bus Creator3/2  "SEL751-01_LogicTrip"
  [SEL751_ScaledSignals] -> SEL751_DigitalAnalog_IO_OpBlocks/1(SEL751-01_ScaledSignals)
  Memory/1 -> HWCtrl_Outputs/1

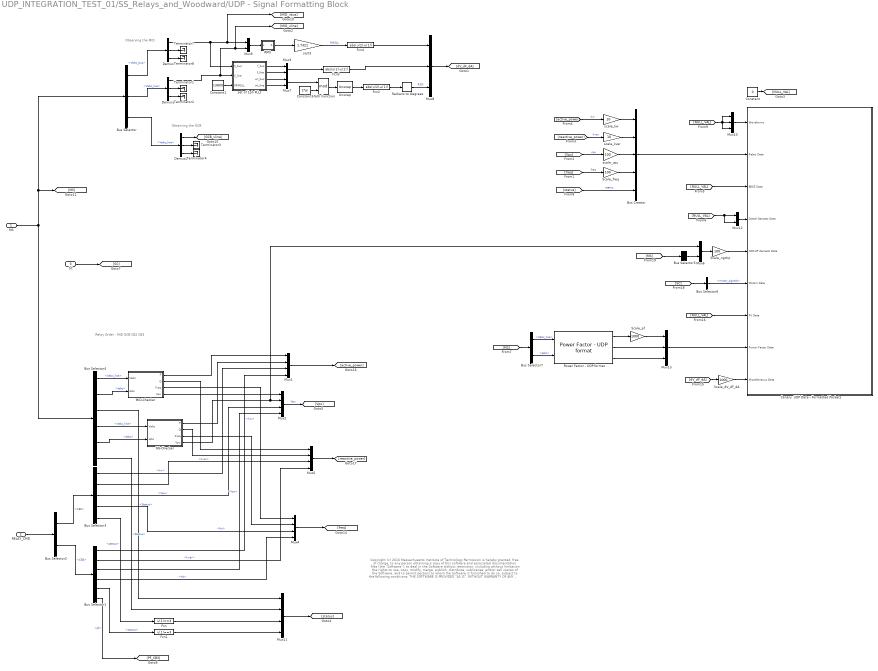
== system UDP_INTEGRATION_TEST_01/SS_Relays_and_Woodward/UDP - Signal Formatting Block ==
  note: Observing the MID
  note: Relay Order :
      | MID
      | GCB
      | CB2
      | CB3
  note: Observing the GCB
  note: Copyright (c) 2016 Massachusetts Institute of Technology
      | Permission is hereby granted, free of charge, to any person obtaining a copy of this software and associated documentation files (the "Software"), to deal
      | in the Software without restriction, including without limitation the rights to use, copy, modify, merge, publish, distribute, sublicense, and/or sell copies of the
      | Software, and to permit persons to whom the Software is furnished to do so, subject to the following conditions:
      |
      | THE SOFTWARE IS PROVIDED "AS IS", WITHOUT WARRANTY OF ANY KIND, EXPRESS OR IMPLIED, INCLUDING BUT NOT LIMITED TO THE
      | WARRANTIES OF MERCHANTABILITY, FITNESS FOR A PARTICULAR PURPOSE AND NONINFRINGEMENT. IN NO EVENT SHALL THE AUTHORS
      | OR COPYRIGHT HOLDERS BE LIABLE FOR ANY CLAIM, DAMAGES OR OTHER LIABILITY, WHETHER IN AN ACTION OF CONTRACT, TORT OR
      | OTHERWISE, ARISING FROM, OUT OF OR IN CONNECTION WITH THE SOFTWARE OR THE USE OR OTHER DEALINGS IN THE SOFTWARE
  MS : Inport
  RELAY_CMD : Inport  Port=2
  SC : Inport  Port=3
  Bus Creator : BusCreator  Inputs=5
  Bus Selector : BusSelector  OutputSignals=MID.Vabc_bus,MID.Vabc_line,NG_CHP_MS.NG_CHP_GCB.Vabc_line
  Bus Selector1 : BusSelector  OutputSignals=m.kw,m.kvar,m.Vpu,m.Hz,m.status,m.pf
  Bus Selector2 : BusSelector  OutputSignals=CB2,CB3
  Bus Selector3 : BusSelector  OutputSignals=m.kw,m.kvar,m.Vpu,m.Hz,m.status
  Bus Selector4 : BusSelector  OutputSignals=MID.Vabc_line,MID.Iabc,MID.Status,NG_CHP_MS.NG_CHP_GCB.Vabc_line,NG_CHP_MS.NG_CHP_GCB.Iabc,NG_CHP_MS.NG_CHP_GCB.Status
  Bus Selector5 : BusSelector  OutputSignals=NG_CHP_MS.CHPData.TempActual,NG_CHP_MS.CHPData.Thermal data.Heat Recovered; MBtu/hr,NG_CHP_MS.CHPData.Thermal data.Nm^3 per hour NG fuel usage,NG_CHP_MS.CHPData.Thermal data.lbm/hr NOx,NG_CHP_MS.CHPData.Thermal data.CO2 lbm/hr,NG_CHP_MS.CHPData.HeatFromBoiler MBtu/hr,NG_CHP_MS.CHPData.CHPHeatContribution MBtu/hr  OutputAsBus=on
  Bus Selector6 : BusSelector  OutputSignals=motor_signals
  Bus Selector7 : BusSelector  OutputSignals=MID.Vabc_line,MID.Iabc
  Canary  UDP Data - Formatted Packets : Subsystem  mask(UDP Data Block){ProfileID=3, NumOfWaveforms=[0,1,1], NumOfRelays=[4, [10, 10, 100, 100]], NumOfBatteries=0, NumOfDieselGensets=[0,1], NumOfNGCHPGensets=[1, [100, 100, 100, 100, 100, 100, 100, 100]], NumOfMotors=1, NumOfPVs=0, NumOfPF=[1, [1000]], NumOfMiscellaneousDataScales=1, NumOfMiscellaneousDataSignalsScales=[[3, 1000]]}
      mask prompts: ProfileID "Profile ID"; NumOfWaveforms "Waveform Data"; NumOfRelays "Relay Data"; NumOfBatteries "# of Batteries"; NumOfDieselGensets "Diesel Gensets Data"; NumOfNGCHPGensets "NG-CHP Gensets Data"; NumOfMotors "# of Motors"; NumOfPVs "# of PVs"; NumOfPF "Power Factor Data"; NumOfMiscellaneousDataScales "Misc. Data - No. of Scale Factors"; NumOfMiscellaneousDataSignalsScales "Misc. - No. Signals and Scale Values"
      mask help:
      | * All signal scaling/modifications should be external to this block
      |
      | Profile ID: (1-Sheriff, 2-Banshee, 3-Canary, 4-Siren)
      |
      | Waveforms Data: No. of per phase waveforms sent at 5Hz rate, point per waveforms [dt=80us, 208; dt=100us, 166], and scaling factor.
      | -Input format: [No. of waveforms, No. of datapoints, scale]
      | -Ex. for Canary:[3, 166, 100]
      |
      | Relay Data: No. of relays feeding packet data to breakers in display - mapped/indexed in ascending order
      | -Packet order: Active power(kW), reactive power(kVAR), voltage(per-unit), frequency (Hz), breaker status (1:closed, 0:open)
      | -Input format: [No. of Relays, [scale_kW, scale_kVAR, scale_Vpu, scale_Hz]]
      | -Ex. for Canary:[4, [10, 10, 100, 100]]
      |
      | No. of Batteries: TBD
      | -Ex. for Canary: [0]
      |
      | No. of Diesel Gensets: No. of diesel gensets in the system feeding data to the display.
      | -Packet order: Fuel comsumption (Gals/hr), terminal voltage(per-unit)
      | -Input format: [No. of gensets, [scale_fuel, scale_Vpu]]
      | -Ex. for Canary: [0, [1,1]]
      |
      | No. of NG/CHP Gensets: TBD
      | -Ex. for Canary: [0]
      |
      | Motors Data: No. of motors monitored in the system. Currently, only looking at motor on/off state.
      | -Input format: [No. of motors]
      | -Ex. for Canary: [1]
      |
      | No. of PV: TBD
      | -Ex. for Canary: [0]
      |
      | Power Factor Data: No. of power factors to be displayed in the system and scale value. The same scale factor will be applied to all power factors.
      | -Packet order: power factor, import/export, lagging/leading
      | -Input format: [No. of Power Factors, scale_pf]
      | -Ex. for Canary:[1, 1000]
      |
      | Misc. Data - No. of Scale factor: No. of scale factors to be applied to each signal-set.
      | -Ex. for Canary: [3]
      |
      | Misc. Data - No. of Signals and Scale Values: Size of signal set and scale value to be applied to the signal-set.
      | -Ex. for Canary: [[1, 1000], [6, 100], [3, 10]]
  Constant : Constant  Value=0
  Constant1 : Constant  Value=13800
  Constant3 : Constant  Value=2*pi
  Demux : Demux  Outputs=3
  Demux1 : Demux  Outputs=3
  Demux2 : Demux  Outputs=3
  Fcn : Fcn  Expr=u(1)==3
  Fcn1 : Fcn  Expr=u(1)==3
  Fcn2 : Fcn  Expr=abs(u(2)-u(1))  SampleTime=Ts
  Fcn3 : Fcn  Expr=abs(u(2)-u(1))  SampleTime=Ts
  Fcn4 : Fcn  Expr=abs(u(2)-u(1))  SampleTime=Ts
  MID-Checker : Subsystem  mask{kv=13.8}
      mask prompts: kv "Base kV"
  Math Function : Math  Operator=mod  SampleTime=Ts  SaturateOnIntegerOverflow=on
  Mux{1..2,4..5,11} (5 alike) : Mux
  Mux10 : Mux  Inputs=3
  Mux{3,6..7,9,12} (5 alike) : Mux  Inputs=2
  Mux13 : Mux  Inputs=3
  Mux8 : Mux  Inputs=3
  NG-Checker : Subsystem  mask{kv=13.8}
      mask prompts: kv "Base kV"
  Power Factor - UDP format : udp_powerfactor_lib/Power Factor - UDP format
  RMS : Subsystem
  Radians to Degrees : simulink_extras/Transformations/Radians to Degrees
  Scale_dV_dF_dA : Gain  Gain=1000
  Scale_freq : Gain  Gain=100
  Scale_ngchp : Gain  Gain=100
  Scale_pf : Gain  Gain=1000
  Terminator{1..4,7..8} (6 alike) : Terminator
  Unwrap : dspsigops/Unwrap  tol=pi  InputProcessing=Columns as channels (frame based)  running=off
  scale_kvar : Gain  Gain=10
  scale_kw : Gain  Gain=10
  scale_vpu : Gain  Gain=100
  set of 1ph PLLs : Subsystem
  sqrt3 : Gain  Gain=1.7321
  wires:
  RELAY_CMD/1 -> Bus Selector2/1
  Bus Selector2/2 -> Bus Selector1/1  "<CB3>"
  Bus Selector2/1 -> Bus Selector3/1  "<CB2>"
  Mux2/1 -> [Vpu]  "Vpu"
  Demux/2 -> Terminator7/1
  Demux/3 -> Terminator8/1
  Demux1/2 -> Terminator1/1
  Demux1/3 -> Terminator2/1
  Demux/1 -> [MID_vbus], Mux9/1, set of 1ph PLLs/1(V_bus)
  Demux1/1 -> set of 1ph PLLs/2(V_line), [MID_vline], Mux9/2
  Bus Selector/1 -> Demux/1  "<Vabc_bus>"
  Bus Selector/2 -> Demux1/1  "<Vabc_line>"
  Mux3/1 -> Fcn3/1
  sqrt3/1 -> Fcn4/1  "RMSLL"
  RMS/1(S) -> sqrt3/1
  Math Function/1 -> Unwrap/1
  Mux7/1 -> Math Function/1
  Constant3/1 -> Math Function/2
  set of 1ph PLLs/1(f_bus) -> Mux3/1
  set of 1ph PLLs/2(f_line) -> Mux3/2
  Mux9/1 -> RMS/1(s)
  set of 1ph PLLs/3(wt_bus) -> Mux7/1
  set of 1ph PLLs/4(wt_line) -> Mux7/2
  Mux8/1 -> [dV_dF_dA]
  Constant1/1 -> set of 1ph PLLs/3(VRMSLL)
  Demux2/2 -> Terminator3/1
  Demux2/3 -> Terminator4/1
  Bus Selector/3 -> Demux2/1  "<Vabc_line>"
  Demux2/1 -> [GCB_vline]
  MS/1 -> [MS], Bus Selector/1, Bus Selector4/1
  Bus Selector4/3 -> Mux11/1  "<Status>"
  Bus Selector4/1 -> MID-Checker/1(Vabc)  "<Vabc_line>"
  Bus Selector4/2 -> MID-Checker/2(Iabc)  "<Iabc>"
  Bus Selector1/3 -> Mux2/4  "<Vpu>"
  Bus Selector4/4 -> NG-Checker/1(Vabc)  "<Vabc_line>"
  Bus Selector4/5 -> NG-Checker/2(Iabc)  "<Iabc>"
  MID-Checker/4(Vpu) -> Mux2/1
  NG-Checker/4(Vpu) -> Mux6/1, Mux2/2
  Bus Selector3/2 -> Mux5/3  "<kvar>"
  Bus Selector3/1 -> Mux1/3  "<kw>"
  Bus Selector3/3 -> Mux2/3  "<Vpu>"
  Bus Selector3/4 -> Mux4/3  "<Hz>"
  Bus Selector3/5 -> Fcn/1  "<status>"
  Bus Selector1/4 -> Mux4/4  "<Hz>"
  Bus Selector1/5 -> Fcn1/1  "<status>"
  MID-Checker/1(P) -> Mux1/1
  NG-Checker/1(P) -> Mux1/2
  MID-Checker/2(Q) -> Mux5/1
  NG-Checker/2(Q) -> Mux5/2
  MID-Checker/3(Freq) -> Mux4/1
  NG-Checker/3(Freq) -> Mux4/2
  Bus Selector4/6 -> Mux11/2  "<Status>"
  Mux1/1 -> [active_power]
  Mux5/1 -> [reactive_power]
  Mux4/1 -> [freq]
  Mux11/1 -> [status]
  Fcn1/1 -> Mux11/4
  Fcn/1 -> Mux11/3
  [reactive_power] -> scale_kvar/1  "kvar"
  [Vpu] -> scale_vpu/1  "vpu"
  [freq] -> Scale_freq/1  "freq"
  [status] -> Bus Creator/5  "status"
  Bus Creator/1 -> Canary  UDP Data - Formatted Packets/2(Relay Data)
  Constant/1 -> [NULL_VAL]
  [NULL_VAL] -> Canary  UDP Data - Formatted Packets/3(BESS Data)
  [NULL_VAL] -> Canary  UDP Data - Formatted Packets/7(PV Data)
  SC/1 -> [SC]
  [SC] -> Bus Selector6/1
  Bus Selector6/1 -> Canary  UDP Data - Formatted Packets/6(Motors Data)  "<motor_signals>"
  Power Factor - UDP format/1 -> Scale_pf/1
  Mux6/1 -> Scale_ngchp/1
  [active_power] -> scale_kw/1  "kw"
  Bus Selector1/6 -> [PF_CB3]  "<pf>"
  Bus Selector1/2 -> Mux5/4  "<kvar>"
  Bus Selector1/1 -> Mux1/4  "<kw>"
  scale_kw/1 -> Bus Creator/1
  scale_kvar/1 -> Bus Creator/2
  Scale_freq/1 -> Bus Creator/4
  scale_vpu/1 -> Bus Creator/3
  Radians to Degrees/1 -> Mux8/3  "R2D"
  Unwrap/1 -> Fcn2/1
  Scale_pf/1 -> Mux13/1
  [MS] -> Bus Selector7/1
  Bus Selector7/1 -> Power Factor - UDP format/1  "<Vabc_line>"
  Bus Selector7/2 -> Power Factor - UDP format/2  "<Iabc>"
  Power Factor - UDP format/2 -> Mux13/2
  Power Factor - UDP format/3 -> Mux13/3
  Mux13/1 -> Canary  UDP Data - Formatted Packets/8(Power Factor Data)
  Fcn3/1 -> Mux8/2
  Fcn4/1 -> Mux8/1
  Fcn2/1 -> Radians to Degrees/1
  [dV_dF_dA] -> Scale_dV_dF_dA/1
  Scale_dV_dF_dA/1 -> Canary  UDP Data - Formatted Packets/9(Miscellaneous Data)
  [MS] -> Bus Selector5/1
  Scale_ngchp/1 -> Canary  UDP Data - Formatted Packets/5(NGCHP Gensets Data)
  Bus Selector5/1 -> Mux6/2
  Mux10/1 -> Canary  UDP Data - Formatted Packets/1(Waveforms)
  [NULL_VAL] -> Mux10/3, Mux10/1, Mux10/2
  Mux12/1 -> Canary  UDP Data - Formatted Packets/4(Diesel Gensets Data)
  [NULL_VAL] -> Mux12/2, Mux12/1

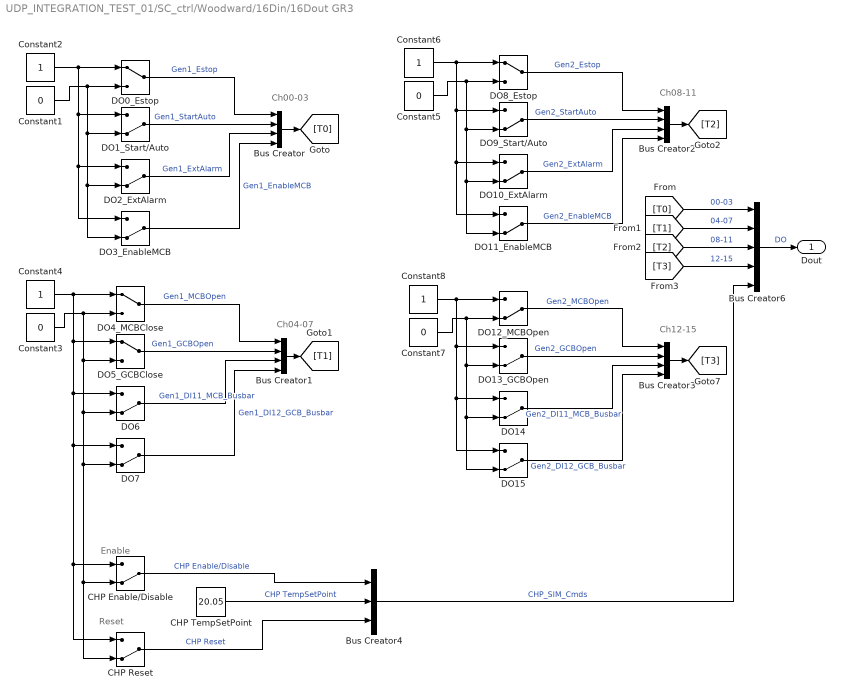
== system UDP_INTEGRATION_TEST_01/SC_ctrl/Woodward/16Din/16Dout GR3 ==
  note: Reset
  note: Enable
  note: Ch12-15
  note: Ch08-11
  note: Ch04-07
  note: Ch00-03
  Bus Creator{,1..3} (4 alike) : BusCreator
  Bus Creator4 : BusCreator  Inputs=3
  Bus Creator6 : BusCreator  Inputs=5
  CHP Enable/Disable : ManualSwitch  CurrentSetting=0
  CHP Reset : ManualSwitch  CurrentSetting=0
  CHP TempSetPoint : Constant  Value=20.05
  Constant{1,3,5,7} (4 alike) : Constant  Value=0
  Constant{2,4,6,8} (4 alike) : Constant
  DO0_Estop : ManualSwitch
  DO10_ExtAlarm : ManualSwitch  CurrentSetting=0
  DO11_EnableMCB : ManualSwitch  CurrentSetting=0
  DO12_MCBOpen : ManualSwitch  CurrentSetting=0
  DO13_GCBOpen : ManualSwitch  CurrentSetting=0
  DO{6..7,14..15} (4 alike) : ManualSwitch  CurrentSetting=0
  DO1_Start/Auto : ManualSwitch  CurrentSetting=0
  DO2_ExtAlarm : ManualSwitch  CurrentSetting=0
  DO3_EnableMCB : ManualSwitch  CurrentSetting=0
  DO4_MCBClose : ManualSwitch
  DO5_GCBClose : ManualSwitch
  DO8_Estop : ManualSwitch
  DO9_Start/Auto : ManualSwitch  CurrentSetting=0
  Dout : Outport
  wires:
  [T3] -> Bus Creator6/4  "12-15"
  [T2] -> Bus Creator6/3  "08-11"
  [T1] -> Bus Creator6/2  "04-07"
  [T0] -> Bus Creator6/1  "00-03"
  Bus Creator2/1 -> [T2]
  Bus Creator3/1 -> [T3]
  Bus Creator1/1 -> [T1]
  Bus Creator/1 -> [T0]
  DO15/1 -> Bus Creator3/4  "Gen2_DI12_GCB_Busbar"
  DO14/1 -> Bus Creator3/3  "Gen2_DI11_MCB_Busbar"
  DO13_GCBOpen/1 -> Bus Creator3/2  "Gen2_GCBOpen"
  DO12_MCBOpen/1 -> Bus Creator3/1  "Gen2_MCBOpen"
  Constant7/1 -> DO12_MCBOpen/2, DO13_GCBOpen/2, DO15/2, DO14/2
  Constant8/1 -> DO12_MCBOpen/1, DO13_GCBOpen/1, DO15/1, DO14/1
  DO11_EnableMCB/1 -> Bus Creator2/4  "Gen2_EnableMCB"
  DO10_ExtAlarm/1 -> Bus Creator2/3  "Gen2_ExtAlarm"
  DO9_Start/Auto/1 -> Bus Creator2/2  "Gen2_StartAuto"
  DO8_Estop/1 -> Bus Creator2/1  "Gen2_Estop"
  Constant5/1 -> DO10_ExtAlarm/2, DO11_EnableMCB/2, DO9_Start/Auto/2, DO8_Estop/2
  Constant6/1 -> DO10_ExtAlarm/1, DO11_EnableMCB/1, DO9_Start/Auto/1, DO8_Estop/1
  DO7/1 -> Bus Creator1/4  "Gen1_DI12_GCB_Busbar"
  DO6/1 -> Bus Creator1/3  "Gen1_DI11_MCB_Busbar"
  DO5_GCBClose/1 -> Bus Creator1/2  "Gen1_GCBOpen"
  DO4_MCBClose/1 -> Bus Creator1/1  "Gen1_MCBOpen"
  Constant3/1 -> DO4_MCBClose/2, DO5_GCBClose/2, DO7/2, CHP Reset/2, CHP Enable/Disable/2, DO6/2
  Constant4/1 -> DO4_MCBClose/1, DO5_GCBClose/1, CHP Reset/1, CHP Enable/Disable/1, DO7/1, DO6/1
  DO3_EnableMCB/1 -> Bus Creator/4  "Gen1_EnableMCB"
  DO2_ExtAlarm/1 -> Bus Creator/3  "Gen1_ExtAlarm"
  DO1_Start/Auto/1 -> Bus Creator/2  "Gen1_StartAuto"
  DO0_Estop/1 -> Bus Creator/1  "Gen1_Estop"
  Constant1/1 -> DO2_ExtAlarm/2, DO3_EnableMCB/2, DO1_Start/Auto/2, DO0_Estop/2
  Constant2/1 -> DO2_ExtAlarm/1, DO3_EnableMCB/1, DO1_Start/Auto/1, DO0_Estop/1
  Bus Creator6/1 -> Dout/1  "DO"
  CHP Enable/Disable/1 -> Bus Creator4/1  "CHP Enable/Disable"
  CHP TempSetPoint/1 -> Bus Creator4/2  "CHP TempSetPoint"
  CHP Reset/1 -> Bus Creator4/3  "CHP Reset"
  Bus Creator4/1 -> Bus Creator6/5  "CHP_SIM_Cmds"

== system UDP_INTEGRATION_TEST_01/SS_Relays_and_Woodward/HWCtrl/GR1 B AIN (CH00-15) ==
  AnalogIn : rtio_opalrt_common/AnalogIn  CtrlName='OpCtrl'  portNb=1  FcnNos=Slot 1 Module B Subsection 1  size=16  maxcount=8  count=8  numchan=8  sampleTime=0
      settings: AttributesFormatString=%<CtrlName>
  AnalogIn1 : rtio_opalrt_common/AnalogIn  CtrlName='OpCtrl'  portNb=2  FcnNos=Slot 1 Module B Subsection 2  size=16  maxcount=8  count=8  numchan=8  sampleTime=0
      settings: AttributesFormatString=%<CtrlName>
  Mux6 : Mux  Inputs=2
  Terminator2 : Terminator
  Terminator3 : Terminator
  Out1 : Outport
  wires:
  AnalogIn/1 -> Mux6/1
  AnalogIn1/1 -> Mux6/2
  AnalogIn/2 -> Terminator2/1
  AnalogIn1/2 -> Terminator3/1
  Mux6/1 -> Out1/1
